simulink model "pitchrate_demo"  (Simulink 6.0)
settings: Solver=ode45  StartTime=0.0  StopTime=100  RelTol=1e-3
PreLoadFcn:
  | load pitchrate_demo
undefined symbols (not defined in the file or in its folder): Ap, Bp, Cp, Dp, k1, k2, k3, Ts
libraries: srolib x1
settings Model: Creator=ksubbara  LastModifiedBy=rlandy
settings DataIOCC: SignalLoggingName=sigsOut
settings DebuggingCC: CheckExecutionContextPreStartOutputMsg=on  CheckExecutionContextRuntimeOutputMsg=on  SolverPrmCheckMsg=none
settings HardwareCC: TargetUnknown=on
settings ModelReferenceCC: UpdateModelReferenceTargets=IfOutOfDate
settings SFSimCC: SFSimApplyToAllLibs=on  SFSimBuildMode=Incremental

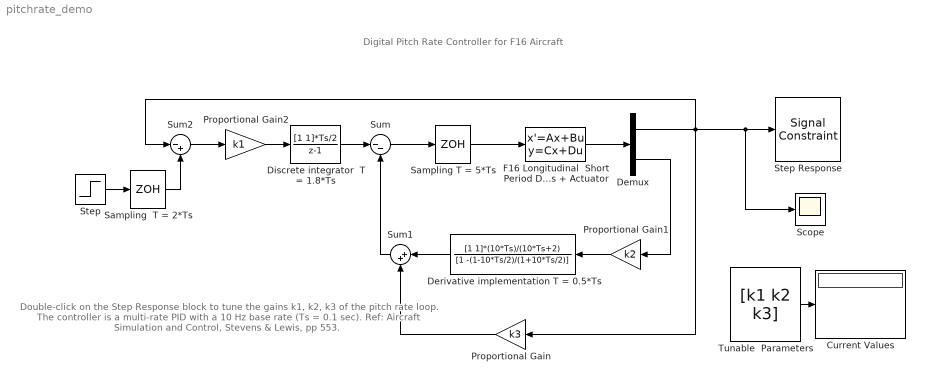
== system pitchrate_demo ==
  note: Digital Pitch Rate Controller for F16 Aircraft
  note: Double-click on the Step Response block to tune
      | the gains k1, k2, k3 of the pitch rate loop.
      |
      | The controller is a multi-rate PID with a
      | 10 Hz base rate (Ts = 0.1 sec).
      |
      | Ref: Aircraft Simulation and Control, Stevens & Lewis, pp 553.
  Current Values : Display
  Demux : Demux  Outputs=2
  Derivative implementation T = 0.5*Ts : DiscreteTransferFcn  Orientation=left  Numerator=[1 1]*(10*Ts)/(10*Ts+2)  Denominator=[1 -(1-10*Ts/2)/(1+10*Ts/2)]  SampleTime=0.4*Ts
  Discrete integrator  T = 1.8*Ts : DiscreteTransferFcn  Numerator=[1 1]*Ts/2  Denominator=[1 -1]  SampleTime=1.8*Ts
  F16 Longitudinal  Short Period Dynamics + Actuator : StateSpace  A=Ap  B=Bp  C=Cp  D=Dp
  Proportional Gain : Gain  Orientation=left  Gain=k3  SaturateOnIntegerOverflow=on
  Proportional Gain1 : Gain  Orientation=left  Gain=k2  SaturateOnIntegerOverflow=on
  Proportional Gain2 : Gain  Gain=k1  SaturateOnIntegerOverflow=on
  Sampling T = 5*Ts : ZeroOrderHold  SampleTime=5*Ts
  Sampling  T = 2*Ts : ZeroOrderHold  SampleTime=2*Ts
  Scope : Scope
  Step : Step  Time=0  SampleTime=0
  Step Response : srolib/Signal Constraint  DialogPosition=[0.04765625 0.298828125 0.378125 0.265625]  SaveIn=workspace  SaveAs=pitchrate_optim  LogID=SRO_DataLog_1  Ylim=[-0.5 1.5]
  Sum : Sum  Inputs=|--  SaturateOnIntegerOverflow=on
  Sum1 : Sum  Orientation=left  Inputs=|++  SaturateOnIntegerOverflow=on
  Sum2 : Sum  Inputs=|-+  SaturateOnIntegerOverflow=on
  Tunable  Parameters : Constant  Value=[k1 k2 k3]
  wires:
  Step/1 -> Sampling  T = 2*Ts/1
  Sampling T = 5*Ts/1 -> F16 Longitudinal  Short Period Dynamics + Actuator/1
  Sum/1 -> Sampling T = 5*Ts/1
  Discrete integrator  T = 1.8*Ts/1 -> Sum/1
  Sum1/1 -> Sum/2
  F16 Longitudinal  Short Period Dynamics + Actuator/1 -> Demux/1
  Proportional Gain/1 -> Sum1/2
  Derivative implementation T = 0.5*Ts/1 -> Sum1/1
  Sampling  T = 2*Ts/1 -> Sum2/2
  Sum2/1 -> Proportional Gain2/1
  Demux/2 -> Proportional Gain1/1
  Tunable  Parameters/1 -> Current Values/1
  Proportional Gain1/1 -> Derivative implementation T = 0.5*Ts/1
  Proportional Gain2/1 -> Discrete integrator  T = 1.8*Ts/1
  Demux/1 -> Proportional Gain/1, Sum2/1, Step Response/1, Scope/1
